simulink model "phase_3"  (R2020b)
settings: Solver=VariableStepAuto  StartTime=0.0  StopTime=10.0  RelTol=1e-3
values from neighbouring files (symbols this model uses):
  A = [0 -pi/16 0;pi/16 0 3*pi/16;0 0 0]    [feedbackControllerFinal.m]
  B = [1/2 1/2;0 0;1/0.15 -1/0.15]    [feedbackControllerFinal.m]
  C = [1 0 0;0 1 0]    [feedbackControllerFinal.m]
  F = -40    [feedbackControllerFinal.m]
  G_closeLoop = inv(C*inv(-(A-B*K1))*B)    [feedbackControllerFinal.m]
  K1 = place(A, B, [-30 -1+4.899*i -1-4.899*i])    [feedbackControllerFinal.m]
  L = L'    [feedbackControllerFinal.m]
  L_R = [1 -400]    [feedbackControllerFinal.m]
  Q1 = [1 0; 0 1; -0.5031 67.9061]    [feedbackControllerFinal.m]
  Q2 = [0 0 6.7909]'    [feedbackControllerFinal.m]
  T = lyap(-F, A, -L_R*C)    [feedbackControllerFinal.m]
settings Model: Creator=BALUCH  LastModifiedBy=BALUCH

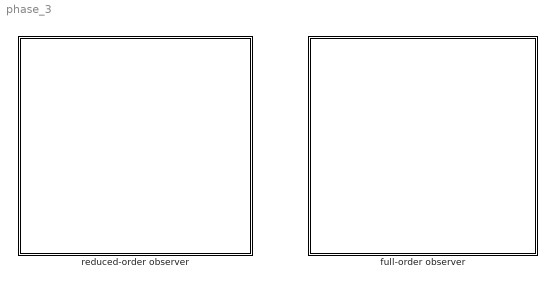
== system phase_3 ==
  "full-order observer " : Subsystem
  reduced-order observer : Subsystem

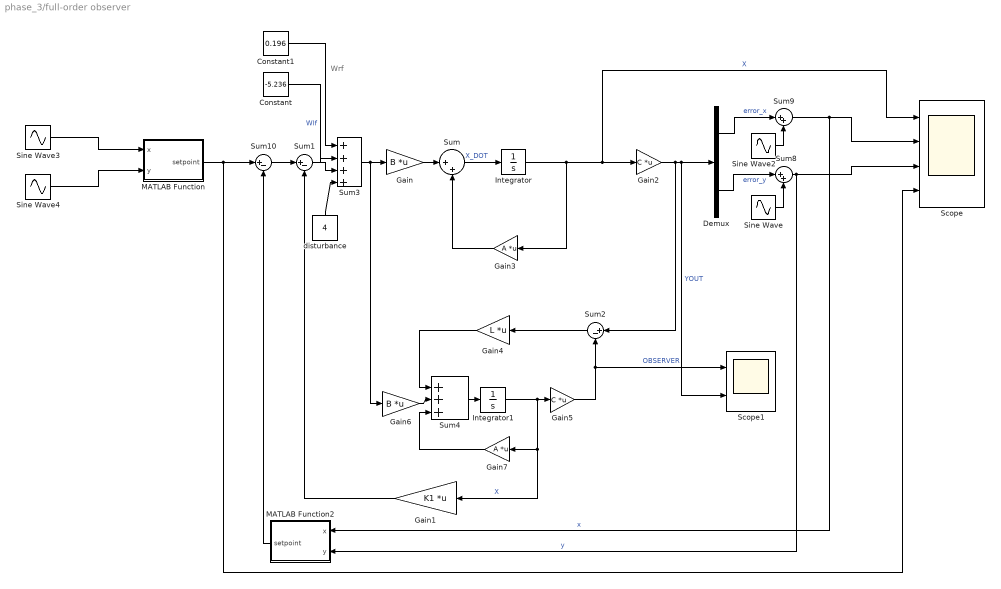
== system phase_3/full-order observer  ==
  note: Wrf
  Constant : Constant  Value=-5.236
  Constant1 : Constant  Value=0.196
  Demux : Demux  Outputs=2
  Gain : Gain  Gain=B  Multiplication=Matrix(K*u)
  Gain1 : Gain  Gain=K1  Multiplication=Matrix(K*u)
  Gain2 : Gain  Gain=C  Multiplication=Matrix(K*u)
  Gain3 : Gain  Gain=A  Multiplication=Matrix(K*u)
  Gain4 : Gain  Gain=L  Multiplication=Matrix(K*u)
  Gain5 : Gain  Gain=C  Multiplication=Matrix(K*u)
  Gain6 : Gain  Gain=B  Multiplication=Matrix(K*u)
  Gain7 : Gain  Gain=A  Multiplication=Matrix(K*u)
  Integrator : Integrator  InitialCondition=[0.1 0.1 0]'
  Integrator1 : Integrator  InitialCondition=[0.4 0.4 0.5]'
  MATLAB Function : MATLAB Function  TreatAsAtomicUnit=on
  MATLAB Function2 : MATLAB Function  TreatAsAtomicUnit=on
  Scope : Scope  NumInputPorts=4
  Scope1 : Scope  NumInputPorts=2
  Sine Wave : Sin  Amplitude=-3  Frequency=pi/16  SampleTime=0
  Sine Wave2 : Sin  Amplitude=3  Frequency=pi/16  Phase=pi/2  SampleTime=0
  Sine Wave3 : Sin  Amplitude=3  Frequency=pi/16  Phase=pi/2  SampleTime=0
  Sine Wave4 : Sin  Amplitude=-3  Frequency=pi/16  SampleTime=0
  Sum : Sum  Inputs=|++
  Sum1 : Sum  Inputs=|+-
  Sum10 : Sum  Inputs=|+-
  Sum2 : Sum  Inputs=|+-
  Sum3 : Sum  Inputs=|++++
  Sum4 : Sum  Inputs=|+++
  Sum8 : Sum  Inputs=|++
  Sum9 : Sum  Inputs=|++
  "disturbance " : Constant  Value=4
  wires:
  Sum8/1 -> MATLAB Function2/2(y), Scope/3  "y"
  Constant/1 -> Sum3/2  "Wlf"
  Sum10/1 -> Sum1/1
  Sine Wave/1 -> Sum8/2
  Integrator/1 -> Gain3/1, Scope/1, Gain2/1  "X"
  Gain1/1 -> Sum1/2
  Demux/1 -> Sum9/1  "error_x"
  "disturbance "/1 -> Sum3/4
  Sum9/1 -> MATLAB Function2/1(x), Scope/2  "x"
  MATLAB Function/1(setpoint) -> Scope/4, Sum10/1
  Constant1/1 -> Sum3/1
  Sine Wave2/1 -> Sum9/2
  Sum3/1 -> Gain6/1, Gain/1
  Gain3/1 -> Sum/2
  Gain2/1 -> Sum2/1, Scope1/2, Demux/1  "YOUT"
  Sum1/1 -> Sum3/3
  Sine Wave3/1 -> MATLAB Function/1(x)
  Gain/1 -> Sum/1
  MATLAB Function2/1(setpoint) -> Sum10/2
  Demux/2 -> Sum8/1  "error_y"
  Sine Wave4/1 -> MATLAB Function/2(y)
  Sum/1 -> Integrator/1  "X_DOT"
  Gain5/1 -> Sum2/2, Scope1/1  "OBSERVER"
  Integrator1/1 -> Gain7/1, Gain1/1, Gain5/1  "X"
  Sum4/1 -> Integrator1/1
  Gain6/1 -> Sum4/2
  Gain4/1 -> Sum4/1
  Gain7/1 -> Sum4/3
  Sum2/1 -> Gain4/1

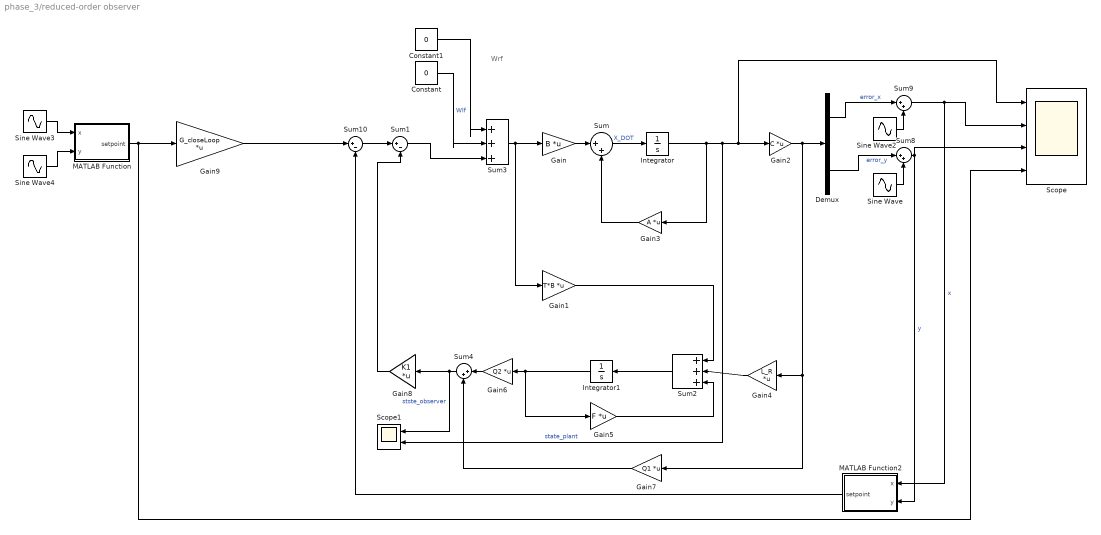
== system phase_3/reduced-order observer ==
  note: Wrf
  Constant : Constant  Value=0
  Constant1 : Constant  Value=0
  Demux : Demux  Outputs=2
  Gain : Gain  Gain=B  Multiplication=Matrix(K*u)
  Gain1 : Gain  Gain=T*B  Multiplication=Matrix(K*u)
  Gain2 : Gain  Gain=C  Multiplication=Matrix(K*u)
  Gain3 : Gain  Gain=A  Multiplication=Matrix(K*u)
  Gain4 : Gain  Gain=L_R  Multiplication=Matrix(K*u)
  Gain5 : Gain  Gain=F  Multiplication=Matrix(K*u)
  Gain6 : Gain  Gain=Q2  Multiplication=Matrix(K*u)
  Gain7 : Gain  Gain=Q1  Multiplication=Matrix(K*u)
  Gain8 : Gain  Gain=K1  Multiplication=Matrix(K*u)
  Gain9 : Gain  Gain=G_closeLoop  Multiplication=Matrix(K*u)
  Integrator : Integrator  InitialCondition=[0.1 0.1 0]'
  Integrator1 : Integrator  InitialCondition=0.05
  MATLAB Function : MATLAB Function  TreatAsAtomicUnit=on
  MATLAB Function2 : MATLAB Function  TreatAsAtomicUnit=on
  Scope : Scope  NumInputPorts=4
  Scope1 : Scope  NumInputPorts=2
  Sine Wave : Sin  Amplitude=-3  Frequency=pi/16  SampleTime=0
  Sine Wave2 : Sin  Amplitude=3  Frequency=pi/16  Phase=pi/2  SampleTime=0
  Sine Wave3 : Sin  Amplitude=3  Frequency=pi/16  Phase=pi/2  SampleTime=0
  Sine Wave4 : Sin  Amplitude=-3  Frequency=pi/16  SampleTime=0
  Sum{,4,8..9} (4 alike) : Sum  Inputs=|++
  Sum1 : Sum  Inputs=|+-
  Sum10 : Sum  Inputs=|+-
  Sum2 : Sum  Inputs=|+++
  Sum3 : Sum  Inputs=|+++
  wires:
  Sum10/1 -> Sum1/1
  Constant/1 -> Sum3/2  "Wlf"
  Sum8/1 -> MATLAB Function2/2(y), Scope/3  "y"
  Sine Wave3/1 -> MATLAB Function/1(x)
  Sine Wave/1 -> Sum8/2
  Sum/1 -> Integrator/1  "X_DOT"
  Sine Wave4/1 -> MATLAB Function/2(y)
  Integrator/1 -> Gain3/1, Scope1/2, Scope/1, Gain2/1  "state_plant"
  Gain2/1 -> Gain7/1, Gain4/1, Demux/1
  Demux/2 -> Sum8/1  "error_y"
  Demux/1 -> Sum9/1  "error_x"
  Gain3/1 -> Sum/2
  MATLAB Function2/1(setpoint) -> Sum10/2
  Gain/1 -> Sum/1
  Sum9/1 -> MATLAB Function2/1(x), Scope/2  "x"
  Sum1/1 -> Sum3/3
  Sum3/1 -> Gain1/1, Gain/1
  Sine Wave2/1 -> Sum9/2
  Constant1/1 -> Sum3/1
  Sum2/1 -> Integrator1/1
  Gain5/1 -> Sum2/3
  Integrator1/1 -> Gain5/1, Gain6/1
  Gain4/1 -> Sum2/2
  Gain1/1 -> Sum2/1
  Gain6/1 -> Sum4/1
  Gain7/1 -> Sum4/2
  Sum4/1 -> Scope1/1, Gain8/1  "stste_observer"
  Gain8/1 -> Sum1/2
  MATLAB Function/1(setpoint) -> Scope/4, Gain9/1
  Gain9/1 -> Sum10/1

== matlab function phase_3/full-order observer /MATLAB Function2 ==
  data: x input; setpoint output; y input
function setpoint = fcn(x, y)

setpoint = [x; y];

== matlab function phase_3/reduced-order observer/MATLAB Function ==
  data: x input; setpoint output; y input
function setpoint = fcn(x, y)

setpoint = [x; y];

== matlab function phase_3/reduced-order observer/MATLAB Function2 ==
  data: x input; setpoint output; y input
function setpoint = fcn(x, y)

setpoint = [x; y];

== matlab function phase_3/full-order observer /MATLAB Function ==
  data: x input; setpoint output; y input
function setpoint = fcn(x, y)

setpoint = [x; y];
